simulink model "ModeInputHandle"  (R2018b)
settings: Solver=FixedStepDiscrete  StartTime=0.0  StopTime=10.0  FixedStep=0.01  RelTol=1e-3
undefined symbols (not defined in the file or in its folder): c, CmprtMdHMIReqExt2Tp1, CmprtMdHMIReqExtTp1, CmprtMdHMIReqTp1, d, e, EZESwReq1, f, g, IfVeSMSeStNumConfig, j, KeSMSuButtonLongPressedThrshldTm_Val, KeSMSuFoldType_Val, KeSMSwSeatSMSSeatMdTrigGapTimer_Val, KeSMSwSeatTrigWaitTimer_Val, KeSMSwSRSActiveValidTm_Val, LckUlckActvtFunc1, LstLckFunc1, LugSelectSw1, MdReqTp1, PowerMode1, SeatOccupiedSts1, SRSMode1, StPassCmprtMdCtrl_Md10_VCUConfig_Val, StPassCmprtMdCtrl_Md11_VCUConfig_Val, StPassCmprtMdCtrl_Md12_VCUConfig_Val, StPassCmprtMdCtrl_Md13_VCUConfig_Val, StPassCmprtMdCtrl_Md1_VCUConfig_Val, StPassCmprtMdCtrl_Md27_VCUConfig_Val, StPassCmprtMdCtrl_Md28_VCUConfig_Val, StPassCmprtMdCtrl_Md29_VCUConfig_Val, StPassCmprtMdCtrl_Md2_VCUConfig_Val, StPassCmprtMdCtrl_Md30_VCUConfig_Val, StPassCmprtMdCtrl_Md31_VCUConfig_Val, StPassCmprtMdCtrl_Md32_VCUConfig_Val, StPassCmprtMdCtrl_Md3_VCUConfig_Val, StPassCmprtMdCtrl_Md53_VCUConfig_Val, StPassCmprtMdCtrl_Md56_VCUConfig_Val, StPassCmprtMdCtrl_Md57_VCUConfig_Val, StPassCmprtMdCtrl_Md58_VCUConfig_Val, StPassCmprtMdCtrl_Md61_VCUConfig_Val, StPassCmprtMdCtrl_Md62_VCUConfig_Val, StPassCmprtMdCtrl_Md8_VCUConfig_Val, StPassCmprtMdCtrl_Md9_VCUConfig_Val, StSrv_StMd10_Config_Val, StSrv_StMd11_Config_Val, StSrv_StMd12_Config_Val, StSrv_StMd13_Config_Val, StSrv_StMd1_Config_Val, StSrv_StMd27_Config_Val, StSrv_StMd28_Config_Val, StSrv_StMd29_Config_Val, StSrv_StMd2_Config_Val, StSrv_StMd30_Config_Val, StSrv_StMd31_Config_Val, StSrv_StMd32_Config_Val, StSrv_StMd3_Config_Val, StSrv_StMd8_Config_Val, StSrv_StMd9_Config_Val, VehMovState1
libraries: MSMLib x91
(part 9 of 9)

== stateflow chart ModeInputHandle/ModelInputHandleRunnable_sys/Subsystem1/AcsEntry4s2RMdReq /ButtonLongPressed2/Chart1 ==
  state NotPressed
    en:
    oMdReq = false;
  state ButtonPressed
    state idle
    state idle1
      en:
      oMdReq = true;
    (default) -> idle
    idle -> idle1 : [after(iLongPressThrshhldTm,tick)]
  (default) -> NotPressed : {oMdInterruptCnt = 0;}
  NotPressed -> NotPressed [order 1] : [(iSRSMode != SRSCurMode1.SRSMode_None) &&...
      | hasChangedTo(iCnfmSwReq, true)]
      | {oMdInterruptCnt ++;}
  NotPressed -> ButtonPressed [order 2] : [iCurMdState == MdTp1.MdTp_None &&...
      | hasChangedTo(iSrc, true)]
  ButtonPressed -> NotPressed : [!iSrc]
  data: iSrc input boolean; oMdReq output boolean; oMdInterruptCnt output uint8; iLongPressThrshhldTm input uint8; iCurMdState input Enum: MdTp1; iCmpReq input; iCnfmSwReq input boolean; iSRSMode input Enum: SRSCurMode1

== stateflow chart ModeInputHandle/ModelInputHandleRunnable_sys/Subsystem1/AcsEntry4s2RMdReq /ButtonLongPressed/Chart1 ==
  state NotPressed
    en:
    oMdReq = false;
  state ButtonPressed
    state idle
      en:
      oMdInterruptCnt ++;
    state idle1
      en:
      oMdReq=true;
    (default) -> idle
    idle -> idle1 [order 1] : [after(iLongPressThrshhldTm,tick)]
  state wait
    en:
    oMdReq = false;
  (default) -> NotPressed : {oMdInterruptCnt = 0;}
  NotPressed -> ButtonPressed : [hasChangedTo(iSrc, true)]
  idle -> NotPressed [order 2] : [!iSrc]
  idle1 -> wait [order 2] : [after(5,tick)]
      | //[after(2,tick)]
  wait -> NotPressed : [!iSrc]
  idle1 -> NotPressed [order 1] : [!iSrc]
  data: iSrc input boolean; oMdReq output boolean; oMdInterruptCnt output uint8; iLongPressThrshhldTm input uint8

== stateflow chart ModeInputHandle/ModelInputHandleRunnable_sys/Subsystem1/AcsExit4s2RMdReq/ButtonLongPressed/Chart1 ==
  state NotPressed
    en:
    oMdReq = false;
  state ButtonPressed
    state idle
      en:
      oMdInterruptCnt ++;
    state idle1
      en:
      oMdReq=true;
    (default) -> idle
    idle -> idle1 [order 1] : [after(iLongPressThrshhldTm,tick)]
  state wait
    en:
    oMdReq = false;
  (default) -> NotPressed : {oMdInterruptCnt = 0;}
  NotPressed -> ButtonPressed : [hasChangedTo(iSrc, true)]
  idle -> NotPressed [order 2] : [!iSrc]
  idle1 -> wait [order 2] : [after(5,tick)]
      | //[after(2,tick)]
  wait -> NotPressed : [!iSrc]
  idle1 -> NotPressed [order 1] : [!iSrc]
  data: iSrc input boolean; oMdReq output boolean; oMdInterruptCnt output uint8; iLongPressThrshhldTm input uint8

== stateflow chart ModeInputHandle/ModelInputHandleRunnable_sys/Subsystem1/AcsExit4s2RMdReq/ButtonLongPressed2/Chart1 ==
  state NotPressed
    en:
    oMdReq = false;
  state ButtonPressed
    state idle
    state idle1
      en:
      oMdReq = true;
    (default) -> idle
    idle -> idle1 : [after(iLongPressThrshhldTm,tick)]
  (default) -> NotPressed : {oMdInterruptCnt = 0;}
  NotPressed -> NotPressed [order 1] : [(iSRSMode != SRSCurMode1.SRSMode_None) &&...
      | hasChangedTo(iCnfmSwReq, true)]
      | {oMdInterruptCnt ++;}
  NotPressed -> ButtonPressed [order 2] : [iCurMdState == MdTp1.MdTp_None &&...
      | hasChangedTo(iSrc, true)]
  ButtonPressed -> NotPressed : [!iSrc]
  data: iSrc input boolean; oMdReq output boolean; oMdInterruptCnt output uint8; iLongPressThrshhldTm input uint8; iCurMdState input Enum: MdTp1; iCmpReq input; iCnfmSwReq input boolean; iSRSMode input Enum: SRSCurMode1

== stateflow chart ModeInputHandle/ModelInputHandleRunnable_sys/Subsystem1/AcsEntryMdReq/ButtonLongPressed1/Chart1 ==
  state NotPressed
    en:
    oMdReq = false;
  state ButtonPressed
    state idle
      en:
      oMdInterruptCnt ++;
    state idle1
      en:
      oMdReq=true;
    (default) -> idle
    idle -> idle1 [order 1] : [after(iLongPressThrshhldTm,tick)]
  state wait
    en:
    oMdReq = false;
  (default) -> NotPressed : {oMdInterruptCnt = 0;}
  NotPressed -> ButtonPressed : [hasChangedTo(iSrc, true)]
  idle -> NotPressed [order 2] : [!iSrc]
  idle1 -> wait [order 2] : //[after(5,tick)]
      | [after(2,tick)]
  wait -> NotPressed : [!iSrc]
  idle1 -> NotPressed [order 1] : [!iSrc]
  data: iSrc input boolean; oMdReq output boolean; oMdInterruptCnt output uint8; iLongPressThrshhldTm input uint8

== stateflow chart ModeInputHandle/ModelInputHandleRunnable_sys/Subsystem1/AcsEntryAll4sBwdMdReq/Chart ==
  state UpdateOcclastStat [function]
    (default) -> (junction 55)
    (junction 55) -> (junction 57) [order 1] : [hasChanged(iNotSecRowLeSeaOccStat)]
    (junction 55) -> (junction 62) [order 2]
    (junction 57) -> (junction 59) : {iNotSecRowLeSeaOccStat_last = iNotSecRowLeSeaOccStat;}
    (junction 59) -> (junction 62)
    (junction 62) -> (junction 61)
    (junction 61) -> (junction 65) [order 1] : [hasChanged(iNotSecRowRtSeaOccStat)]
    (junction 61) -> (junction 70) [order 2]
    (junction 65) -> (junction 68) : {iNotSecRowRtSeaOccStat_last = iNotSecRowRtSeaOccStat;}
    (junction 68) -> (junction 70)
    (junction 70) -> (junction 73)
  state Wait1
    du:
    UpdateOcclastStat();
  state active
    en:
    oReq = true;
    iNotSecRowLeSeaOccStat_last = iNotSecRowLeSeaOccStat;
    iNotSecRowRtSeaOccStat_last = iNotSecRowRtSeaOccStat;
    du:
    UpdateOcclastStat();
  state inactive
    en:
    oReq = false;
    iNotSecRowLeSeaOccStat_last = iNotSecRowLeSeaOccStat;
    iNotSecRowRtSeaOccStat_last = iNotSecRowRtSeaOccStat;
    du:
    UpdateOcclastStat();
  state Wait2
    du:
    UpdateOcclastStat();
  (default) -> inactive
  inactive -> Wait1 [order 1] : [hasChangedTo(iRLDoorAjarSwAct,false)&&(iRRDoorAjarSwAct == false)]
  inactive -> Wait1 [order 2] : [hasChangedTo(iRRDoorAjarSwAct,false)&&(iRLDoorAjarSwAct == false)]
  Wait1 -> active [order 3] : [(((iNotSecRowLeSeaOccStat == SeatOccupiedSts1.SeatOccupiedSts_Occupied)&&...
      | (iNotSecRowLeSeaOccStat_last == SeatOccupiedSts1.SeatOccupiedSts_Empty))||...
      |  ((iNotSecRowRtSeaOccStat == SeatOccupiedSts1.SeatOccupiedSts_Occupied)&&...
      | (iNotSecRowRtSeaOccStat_last == SeatOccupiedSts1.SeatOccupiedSts_Empty)))]
  inactive -> Wait1 [order 4] : [hasChangedTo(iRLDoorAjarSwAct,false)&&hasChangedTo(iRRDoorAjarSwAct,false)]
  Wait1 -> inactive [order 1] : [after(iKeSMSwSeatSMSSeatMdTrigGapTimer,tick)]
  Wait1 -> inactive [order 2] : [(iRLDoorAjarSwAct == true)||(iRRDoorAjarSwAct == true)]
  Wait2 -> active [order 3] : [hasChangedTo(iRLDoorAjarSwAct,false) && (iRRDoorAjarSwAct == false)]
  Wait2 -> active [order 4] : [hasChangedTo(iRRDoorAjarSwAct,false) && (iRLDoorAjarSwAct == false)]
  inactive -> Wait2 [order 3] : [((iNotSecRowLeSeaOccStat == SeatOccupiedSts1.SeatOccupiedSts_Occupied)&&...
      | (iNotSecRowLeSeaOccStat_last == SeatOccupiedSts1.SeatOccupiedSts_Empty))||...
      |  ((iNotSecRowRtSeaOccStat == SeatOccupiedSts1.SeatOccupiedSts_Occupied)&&...
      | (iNotSecRowRtSeaOccStat_last == SeatOccupiedSts1.SeatOccupiedSts_Empty))]
  Wait2 -> active [order 5] : [hasChangedTo(iRLDoorAjarSwAct,false)&&hasChangedTo(iRRDoorAjarSwAct,false)]
  Wait2 -> inactive [order 1] : [after(iKeSMSwSeatSMSSeatMdTrigGapTimer,tick)]
  Wait2 -> inactive [order 2] : [(iNotSecRowLeSeaOccStat == SeatOccupiedSts1.SeatOccupiedSts_Empty)&&...
      | (iNotSecRowRtSeaOccStat == SeatOccupiedSts1.SeatOccupiedSts_Empty)]
  active -> inactive : [after(3,tick)]
  data: oReq output boolean; iRLDoorAjarSwAct input boolean; iRRDoorAjarSwAct input boolean; iKeSMSwSeatSMSSeatMdTrigGapTimer input uint16; iNotSecRowLeSeaOccStat input Enum: SeatOccupiedSts1; iNotSecRowRtSeaOccStat input Enum: SeatOccupiedSts1; iNotSecRowLeSeaOccStat_last local Enum: SeatOccupiedSts1 size=1; iNotSecRowRtSeaOccStat_last local Enum: SeatOccupiedSts1 size=1; flag local uint8 size=1

== stateflow chart ModeInputHandle/ModelInputHandleRunnable_sys/Subsystem1/AcsEntryAll4sFwdMdReq/Chart ==
  state Init
    en:
    AcsEntryAll4sFwdMdV = false;
  state WaitOccSign
    en:
    AcsEntryAll4sFwdMdV = false;
  state MdAvail
    en:
    AcsEntryAll4sFwdMdV = true;
  (default) -> Init
  WaitOccSign -> Init [order 2] : [after(iKeSMSwSeatTrigWaitTimer,tick)]
  (junction 34) -> WaitOccSign [order 2]
  WaitOccSign -> MdAvail [order 1] : [(ibVehMovState == true) && (ibSysPwrMd == true) &&...
      | (ibNotSecRowLRSeaOccEmpty == true)]
  Init -> (junction 34) : [(ibLstLckFunc == true) && (ibLstLckChange == true) &&...
      |  (ibLckUlckActvtFunc == true)]
  (junction 34) -> MdAvail [order 1] : [(ibVehMovState == true) && (ibSysPwrMd == true) &&...
      | (ibNotSecRowLRSeaOccEmpty == true)]
  MdAvail -> Init : [(ibVehMovState == false) || (ibSysPwrMd == false) ||...
      |  (ibLstLckFunc == false) || (ibLstLckChange == false) ||...
      |  (ibLckUlckActvtFunc == false) || (ibNotSecRowLRSeaOccEmpty == false)]
  data: ibVehMovState input; ibSysPwrMd input; ibLstLckFunc input; ibLstLckChange input; ibLckUlckActvtFunc input; ibNotSecRowLRSeaOccEmpty input; iKeSMSwSeatTrigWaitTimer input; AcsEntryAll4sFwdMdV output boolean

== stateflow chart ModeInputHandle/ModelInputHandleRunnable_sys/Subsystem1/PasReclinerEntryMdReq/ButtonLongPressed/Chart1 ==
  state NotPressed
    en:
    oMdReq = false;
  state ButtonPressed
    state idle
      en:
      oMdInterruptCnt ++;
    state idle1
      en:
      oMdReq=true;
    (default) -> idle
    idle -> idle1 [order 1] : [after(iLongPressThrshhldTm,tick)]
  state wait
    en:
    oMdReq = false;
  (default) -> NotPressed : {oMdInterruptCnt = 0;}
  NotPressed -> ButtonPressed : [hasChangedTo(iSrc, true)]
  idle -> NotPressed [order 2] : [!iSrc]
  wait -> NotPressed : [!iSrc]
  idle1 -> wait [order 2] : //[after(5,tick)]
      | [after(2,tick)]
  idle1 -> NotPressed [order 1] : [!iSrc]
  data: iSrc input boolean; oMdReq output boolean; oMdInterruptCnt output uint8; iLongPressThrshhldTm input uint8

== stateflow chart ModeInputHandle/ModelInputHandleRunnable_sys/Subsystem1/PasReclinerExitMdReq/ButtonLongPressed/Chart1 ==
  state NotPressed
    en:
    oMdReq = false;
  state ButtonPressed
    state idle
      en:
      oMdInterruptCnt ++;
    state idle1
      en:
      oMdReq=true;
    (default) -> idle
    idle -> idle1 [order 1] : [after(iLongPressThrshhldTm,tick)]
  state wait
    en:
    oMdReq = false;
  (default) -> NotPressed : {oMdInterruptCnt = 0;}
  NotPressed -> ButtonPressed : [hasChangedTo(iSrc, true)]
  idle -> NotPressed [order 2] : [!iSrc]
  wait -> NotPressed : [!iSrc]
  idle1 -> wait [order 2] : //[after(5,tick)]
      | [after(2,tick)]
  idle1 -> NotPressed [order 1] : [!iSrc]
  data: iSrc input boolean; oMdReq output boolean; oMdInterruptCnt output uint8; iLongPressThrshhldTm input uint8

== stateflow chart ModeInputHandle/ModelInputHandleRunnable_sys/Subsystem1/UnfoldMdReq/ButtonLongPressed/Chart1 ==
  state NotPressed
    en:
    oMdReq = false;
  state ButtonPressed
    state idle
      en:
      oMdInterruptCnt ++;
    state idle1
      en:
      oMdReq=true;
    (default) -> idle
    idle -> idle1 [order 1] : [after(iLongPressThrshhldTm,tick)]
  state wait
    en:
    oMdReq = false;
  (default) -> NotPressed : {oMdInterruptCnt = 0;}
  NotPressed -> ButtonPressed : [hasChangedTo(iSrc, true)]
  idle -> NotPressed [order 2] : [!iSrc]
  wait -> NotPressed : [!iSrc]
  idle1 -> wait [order 2] : //[after(5,tick)]
      | [after(2,tick)]
  idle1 -> NotPressed [order 1] : [!iSrc]
  data: iSrc input boolean; oMdReq output boolean; oMdInterruptCnt output uint8; iLongPressThrshhldTm input uint8

== stateflow chart ModeInputHandle/ModelInputHandleRunnable_sys/Subsystem1/UnfoldMdReq/ButtonLongPressed1/Chart1 ==
  state NotPressed
    en:
    oMdReq = false;
  state ButtonPressed
    state idle
      en:
      oMdInterruptCnt ++;
    state idle1
      en:
      oMdReq=true;
    (default) -> idle
    idle -> idle1 [order 1] : [after(iLongPressThrshhldTm,tick)]
  state wait
    en:
    oMdReq = false;
  (default) -> NotPressed : {oMdInterruptCnt = 0;}
  NotPressed -> ButtonPressed : [hasChangedTo(iSrc, true)]
  idle -> NotPressed [order 2] : [!iSrc]
  wait -> NotPressed : [!iSrc]
  idle1 -> wait [order 2] : //[after(5,tick)]
      | [after(2,tick)]
  idle1 -> NotPressed [order 1] : [!iSrc]
  data: iSrc input boolean; oMdReq output boolean; oMdInterruptCnt output uint8; iLongPressThrshhldTm input uint8

== stateflow chart ModeInputHandle/ModelInputHandleRunnable_sys/Subsystem1/AcsEntryMdReq/ButtonLongPressed4/Chart1 ==
  state NotPressed
    en:
    oMdReq = false;
  state ButtonPressed
    state idle
      en:
      oMdInterruptCnt ++;
    state idle1
      en:
      oMdReq=true;
    (default) -> idle
    idle -> idle1 [order 1] : [after(iLongPressThrshhldTm,tick)]
  state wait
    en:
    oMdReq = false;
  (default) -> NotPressed : {oMdInterruptCnt = 0;}
  NotPressed -> ButtonPressed : [hasChangedTo(iSrc, true)]
  idle -> NotPressed [order 2] : [!iSrc]
  idle1 -> wait [order 2] : //[after(5,tick)]
      | [after(2,tick)]
  wait -> NotPressed : [!iSrc]
  idle1 -> NotPressed [order 1] : [!iSrc]
  data: iSrc input boolean; oMdReq output boolean; oMdInterruptCnt output uint8; iLongPressThrshhldTm input uint8

== stateflow chart ModeInputHandle/ModelInputHandleRunnable_sys/Subsystem1/AcsEntryMdReq/ButtonLongPressed2/Chart1 ==
  state NotPressed
    en:
    oMdReq = false;
  state ButtonPressed
    state idle
    state idle1
      en:
      oMdReq = true;
    (default) -> idle
    idle -> idle1 : [after(iLongPressThrshhldTm,tick)]
  (default) -> NotPressed : {oMdInterruptCnt = 0;}
  NotPressed -> NotPressed [order 1] : [(iSRSMode != SRSCurMode1.SRSMode_None) &&...
      | hasChangedTo(iCnfmSwReq, true)]
      | {oMdInterruptCnt ++;}
  NotPressed -> ButtonPressed [order 2] : [iCurMdState == MdTp1.MdTp_None &&...
      | hasChangedTo(iSrc, true)]
  ButtonPressed -> NotPressed : [!iSrc]
  data: iSrc input boolean; oMdReq output boolean; oMdInterruptCnt output uint8; iLongPressThrshhldTm input uint8; iCurMdState input Enum: MdTp1; iCmpReq input; iCnfmSwReq input boolean; iSRSMode input Enum: SRSCurMode1

== stateflow chart ModeInputHandle/ModelInputHandleRunnable_sys/Subsystem1/AcsEntryMdReq/ButtonLongPressed3/Chart1 ==
  state NotPressed
    en:
    oMdReq = false;
  state ButtonPressed
    state idle
      en:
      oMdInterruptCnt ++;
    state idle1
      en:
      oMdReq=true;
    (default) -> idle
    idle -> idle1 [order 1] : [after(iLongPressThrshhldTm,tick)]
  state wait
    en:
    oMdReq = false;
  (default) -> NotPressed : {oMdInterruptCnt = 0;}
  NotPressed -> ButtonPressed : [hasChangedTo(iSrc, true)]
  idle -> NotPressed [order 2] : [!iSrc]
  wait -> NotPressed : [!iSrc]
  idle1 -> wait [order 2] : //[after(5,tick)]
      | [after(2,tick)]
  idle1 -> NotPressed [order 1] : [!iSrc]
  data: iSrc input boolean; oMdReq output boolean; oMdInterruptCnt output uint8; iLongPressThrshhldTm input uint8

== stateflow chart ModeInputHandle/ModelInputHandleRunnable_sys/Subsystem1/AcsExtMdReq/ButtonLongPressed/Chart1 ==
  state ButtonPressed
    state idle
      en:
      oMdInterruptCnt ++;
    state idle1
      en:
      oMdReq=true;
    (default) -> idle
    idle -> idle1 [order 1] : [after(iLongPressThrshhldTm,tick)]
  state NotPressed
    en:
    oMdReq = false;
  state wait
    en:
    oMdReq = false;
  (default) -> NotPressed : {oMdInterruptCnt = 0;}
  NotPressed -> ButtonPressed : [hasChangedTo(iSrc, true)]
  idle -> NotPressed [order 2] : [!iSrc]
  idle1 -> wait [order 2] : [after(5,tick)]
      | //[after(2,tick)]
  wait -> NotPressed : [!iSrc]
  idle1 -> NotPressed [order 1] : [!iSrc]
  data: iSrc input boolean; oMdReq output boolean; oMdInterruptCnt output uint8; iLongPressThrshhldTm input uint8

== stateflow chart ModeInputHandle/ModelInputHandleRunnable_sys/Subsystem1/AcsExtMdReq/ButtonLongPressed1/Chart1 ==
  state NotPressed
    en:
    oMdReq = false;
  state ButtonPressed
    state idle
      en:
      oMdInterruptCnt ++;
    state idle1
      en:
      oMdReq=true;
    (default) -> idle
    idle -> idle1 [order 1] : [after(iLongPressThrshhldTm,tick)]
  state wait
    en:
    oMdReq = false;
  (default) -> NotPressed : {oMdInterruptCnt = 0;}
  NotPressed -> ButtonPressed : [hasChangedTo(iSrc, true)]
  idle -> NotPressed [order 2] : [!iSrc]
  idle1 -> wait [order 2] : [after(5,tick)]
      | //[after(2,tick)]
  wait -> NotPressed : [!iSrc]
  idle1 -> NotPressed [order 1] : [!iSrc]
  data: iSrc input boolean; oMdReq output boolean; oMdInterruptCnt output uint8; iLongPressThrshhldTm input uint8

== stateflow chart ModeInputHandle/ModelInputHandleRunnable_sys/Subsystem1/AcsExtMdReq/ButtonLongPressed2/Chart1 ==
  state NotPressed
    en:
    oMdReq = false;
  state ButtonPressed
    state idle
    state idle1
      en:
      oMdReq = true;
    (default) -> idle
    idle -> idle1 : [after(iLongPressThrshhldTm,tick)]
  (default) -> NotPressed : {oMdInterruptCnt = 0;}
  NotPressed -> NotPressed [order 1] : [(iSRSMode != SRSCurMode1.SRSMode_None) &&...
      | hasChangedTo(iCnfmSwReq, true)]
      | {oMdInterruptCnt ++;}
  NotPressed -> ButtonPressed [order 2] : [iCurMdState == MdTp1.MdTp_None &&...
      | hasChangedTo(iSrc, true)]
  ButtonPressed -> NotPressed : [!iSrc]
  data: iSrc input boolean; oMdReq output boolean; oMdInterruptCnt output uint8; iLongPressThrshhldTm input uint8; iCurMdState input Enum: MdTp1; iCmpReq input; iCnfmSwReq input boolean; iSRSMode input Enum: SRSCurMode1

== stateflow chart ModeInputHandle/ModelInputHandleRunnable_sys/Subsystem1/FamilyMdReq/ButtonLongPressed2/Chart1 ==
  state NotPressed
    en:
    oMdReq = false;
  state ButtonPressed
    state idle
    state idle1
      en:
      oMdReq = true;
    (default) -> idle
    idle -> idle1 : [after(iLongPressThrshhldTm,tick)]
  (default) -> NotPressed : {oMdInterruptCnt = 0;}
  NotPressed -> NotPressed [order 1] : [(iSRSMode != SRSMode1.SRSSlctSwStat_None) &&...
      | hasChangedTo(iCnfmSwReq, true)]
      | {oMdInterruptCnt ++;}
  NotPressed -> ButtonPressed [order 2] : [iCurMdState == MdTp1.MdTp_None &&...
      | hasChangedTo(iSrc, true)]
  ButtonPressed -> NotPressed : [!iSrc]
  data: iSrc input boolean; oMdReq output boolean; oMdInterruptCnt output uint8; iLongPressThrshhldTm input uint8; iCurMdState input Enum: MdTp1; iCmpReq input; iCnfmSwReq input boolean; iSRSMode input Enum: SRSCurMode1

== stateflow chart ModeInputHandle/ModelInputHandleRunnable_sys/Subsystem1/FamilyMdReq/ButtonLongPressed4/Chart1 ==
  state NotPressed
    en:
    oMdReq = false;
  state ButtonPressed
    state idle
    state idle1
      en:
      oMdReq = true;
    (default) -> idle
    idle -> idle1 : [after(iLongPressThrshhldTm,tick)]
  (default) -> NotPressed : {oMdInterruptCnt = 0;}
  NotPressed -> NotPressed [order 1] : [(iSRSMode != SRSMode1.SRSSlctSwStat_None) &&...
      | hasChangedTo(iCnfmSwReq, true)]
      | {oMdInterruptCnt ++;}
  NotPressed -> ButtonPressed [order 2] : [iCurMdState == MdTp1.MdTp_None &&...
      | hasChangedTo(iSrc, true)]
  ButtonPressed -> NotPressed : [!iSrc]
  data: iSrc input boolean; oMdReq output boolean; oMdInterruptCnt output uint8; iLongPressThrshhldTm input uint8; iCurMdState input Enum: MdTp1; iCmpReq input; iCnfmSwReq input boolean; iSRSMode input Enum: SRSCurMode1

== stateflow chart ModeInputHandle/ModelInputHandleRunnable_sys/Subsystem1/IntimacyReq/ButtonLongPressed1/Chart1 ==
  state NotPressed
    en:
    oMdReq = false;
  state ButtonPressed
    state idle
    state idle1
      en:
      oMdReq = true;
    (default) -> idle
    idle -> idle1 : [after(iLongPressThrshhldTm,tick)]
  (default) -> NotPressed : {oMdInterruptCnt = 0;}
  NotPressed -> NotPressed [order 1] : [(iSRSMode != SRSMode1.SRSSlctSwStat_None) &&...
      | hasChangedTo(iCnfmSwReq, true)]
      | {oMdInterruptCnt ++;}
  NotPressed -> ButtonPressed [order 2] : [iCurMdState == MdTp1.MdTp_None &&...
      | hasChangedTo(iSrc, true)]
  ButtonPressed -> NotPressed : [!iSrc]
  data: iSrc input boolean; oMdReq output boolean; oMdInterruptCnt output uint8; iLongPressThrshhldTm input uint8; iCurMdState input Enum: MdTp1; iCmpReq input; iCnfmSwReq input boolean; iSRSMode input Enum: SRSCurMode1

== stateflow chart ModeInputHandle/ModelInputHandleRunnable_sys/Subsystem1/IntimacyReq/ButtonLongPressed4/Chart1 ==
  state NotPressed
    en:
    oMdReq = false;
  state ButtonPressed
    state idle
    state idle1
      en:
      oMdReq = true;
    (default) -> idle
    idle -> idle1 : [after(iLongPressThrshhldTm,tick)]
  (default) -> NotPressed : {oMdInterruptCnt = 0;}
  NotPressed -> NotPressed [order 1] : [(iSRSMode != SRSMode1.SRSSlctSwStat_None) &&...
      | hasChangedTo(iCnfmSwReq, true)]
      | {oMdInterruptCnt ++;}
  NotPressed -> ButtonPressed [order 2] : [iCurMdState == MdTp1.MdTp_None &&...
      | hasChangedTo(iSrc, true)]
  ButtonPressed -> NotPressed : [!iSrc]
  data: iSrc input boolean; oMdReq output boolean; oMdInterruptCnt output uint8; iLongPressThrshhldTm input uint8; iCurMdState input Enum: MdTp1; iCmpReq input; iCnfmSwReq input boolean; iSRSMode input Enum: SRSCurMode1

== stateflow chart ModeInputHandle/ModelInputHandleRunnable_sys/Subsystem1/LgrstLtMdReq/ButtonLongPressed2/Chart1 ==
  state NotPressed
    en:
    oMdReq = false;
  state ButtonPressed
    state idle
    state idle1
      en:
      oMdReq = true;
    (default) -> idle
    idle -> idle1 : [after(iLongPressThrshhldTm,tick)]
  (default) -> NotPressed : {oMdInterruptCnt = 0;}
  NotPressed -> NotPressed [order 1] : [(iSRSMode != SRSMode1.SRSSlctSwStat_None) &&...
      | hasChangedTo(iCnfmSwReq, true)]
      | {oMdInterruptCnt ++;}
  NotPressed -> ButtonPressed [order 2] : [iCurMdState == MdTp1.MdTp_None &&...
      | hasChangedTo(iSrc, true)]
  ButtonPressed -> NotPressed : [!iSrc]
  data: iSrc input boolean; oMdReq output boolean; oMdInterruptCnt output uint8; iLongPressThrshhldTm input uint8; iCurMdState input Enum: MdTp1; iCmpReq input; iCnfmSwReq input boolean; iSRSMode input Enum: SRSCurMode1

== stateflow chart ModeInputHandle/ModelInputHandleRunnable_sys/Subsystem1/LgrstLtMdReq/ButtonLongPressed4/Chart1 ==
  state NotPressed
    en:
    oMdReq = false;
  state ButtonPressed
    state idle
    state idle1
      en:
      oMdReq = true;
    (default) -> idle
    idle -> idle1 : [after(iLongPressThrshhldTm,tick)]
  (default) -> NotPressed : {oMdInterruptCnt = 0;}
  NotPressed -> NotPressed [order 1] : [(iSRSMode != SRSMode1.SRSSlctSwStat_None) &&...
      | hasChangedTo(iCnfmSwReq, true)]
      | {oMdInterruptCnt ++;}
  NotPressed -> ButtonPressed [order 2] : [iCurMdState == MdTp1.MdTp_None &&...
      | hasChangedTo(iSrc, true)]
  ButtonPressed -> NotPressed : [!iSrc]
  data: iSrc input boolean; oMdReq output boolean; oMdInterruptCnt output uint8; iLongPressThrshhldTm input uint8; iCurMdState input Enum: MdTp1; iCmpReq input; iCnfmSwReq input boolean; iSRSMode input Enum: SRSCurMode1

== stateflow chart ModeInputHandle/ModelInputHandleRunnable_sys/Subsystem1/LgrstRtMdReq/ButtonLongPressed2/Chart1 ==
  state NotPressed
    en:
    oMdReq = false;
  state ButtonPressed
    state idle
    state idle1
      en:
      oMdReq = true;
    (default) -> idle
    idle -> idle1 : [after(iLongPressThrshhldTm,tick)]
  (default) -> NotPressed : {oMdInterruptCnt = 0;}
  NotPressed -> NotPressed [order 1] : [(iSRSMode != SRSMode1.SRSSlctSwStat_None) &&...
      | hasChangedTo(iCnfmSwReq, true)]
      | {oMdInterruptCnt ++;}
  NotPressed -> ButtonPressed [order 2] : [iCurMdState == MdTp1.MdTp_None &&...
      | hasChangedTo(iSrc, true)]
  ButtonPressed -> NotPressed : [!iSrc]
  data: iSrc input boolean; oMdReq output boolean; oMdInterruptCnt output uint8; iLongPressThrshhldTm input uint8; iCurMdState input Enum: MdTp1; iCmpReq input; iCnfmSwReq input boolean; iSRSMode input Enum: SRSCurMode1

== stateflow chart ModeInputHandle/ModelInputHandleRunnable_sys/Subsystem1/LgrstRtMdReq/ButtonLongPressed4/Chart1 ==
  state NotPressed
    en:
    oMdReq = false;
  state ButtonPressed
    state idle
    state idle1
      en:
      oMdReq = true;
    (default) -> idle
    idle -> idle1 : [after(iLongPressThrshhldTm,tick)]
  (default) -> NotPressed : {oMdInterruptCnt = 0;}
  NotPressed -> NotPressed [order 1] : [(iSRSMode != SRSMode1.SRSSlctSwStat_None) &&...
      | hasChangedTo(iCnfmSwReq, true)]
      | {oMdInterruptCnt ++;}
  NotPressed -> ButtonPressed [order 2] : [iCurMdState == MdTp1.MdTp_None &&...
      | hasChangedTo(iSrc, true)]
  ButtonPressed -> NotPressed : [!iSrc]
  data: iSrc input boolean; oMdReq output boolean; oMdInterruptCnt output uint8; iLongPressThrshhldTm input uint8; iCurMdState input Enum: MdTp1; iCmpReq input; iCnfmSwReq input boolean; iSRSMode input Enum: SRSCurMode1

== stateflow chart ModeInputHandle/ModelInputHandleRunnable_sys/Subsystem1/LugMdReq/ButtonLongPressed/Chart1 ==
  state NotPressed
    en:
    oMdReq = false;
  state ButtonPressed
    state idle
      en:
      oMdInterruptCnt ++;
    state idle1
      en:
      oMdReq=true;
    (default) -> idle
    idle -> idle1 [order 1] : [after(iLongPressThrshhldTm,tick)]
  state wait
    en:
    oMdReq = false;
  (default) -> NotPressed : {oMdInterruptCnt = 0;}
  NotPressed -> ButtonPressed : [hasChangedTo(iSrc, true)]
  idle -> NotPressed [order 2] : [!iSrc]
  wait -> NotPressed : [!iSrc]
  idle1 -> wait [order 2] : //[after(5,tick)]
      | [after(2,tick)]
  idle1 -> NotPressed [order 1] : [!iSrc]
  data: iSrc input boolean; oMdReq output boolean; oMdInterruptCnt output uint8; iLongPressThrshhldTm input uint8

== stateflow chart ModeInputHandle/ModelInputHandleRunnable_sys/Subsystem1/LugMdReq/ButtonLongPressed1/Chart1 ==
  state NotPressed
    en:
    oMdReq = false;
  state ButtonPressed
    state idle
      en:
      oMdInterruptCnt ++;
    state idle1
      en:
      oMdReq=true;
    (default) -> idle
    idle -> idle1 [order 1] : [after(iLongPressThrshhldTm,tick)]
  state wait
    en:
    oMdReq = false;
  (default) -> NotPressed : {oMdInterruptCnt = 0;}
  NotPressed -> ButtonPressed : [hasChangedTo(iSrc, true)]
  idle -> NotPressed [order 2] : [!iSrc]
  idle1 -> wait [order 2] : //[after(5,tick)]
      | [after(2,tick)]
  wait -> NotPressed : [!iSrc]
  idle1 -> NotPressed [order 1] : [!iSrc]
  data: iSrc input boolean; oMdReq output boolean; oMdInterruptCnt output uint8; iLongPressThrshhldTm input uint8

== stateflow chart ModeInputHandle/ModelInputHandleRunnable_sys/Subsystem1/LugMdReq/ButtonLongPressed2/Chart1 ==
  state NotPressed
    en:
    oMdReq = false;
  state ButtonPressed
    state idle
      en:
      oMdInterruptCnt ++;
    state idle1
      en:
      oMdReq=true;
    (default) -> idle
    idle -> idle1 [order 1] : [after(iLongPressThrshhldTm,tick)]
  state wait
    en:
    oMdReq = false;
  (default) -> NotPressed : {oMdInterruptCnt = 0;}
  NotPressed -> ButtonPressed : [hasChangedTo(iSrc, true)]
  idle -> NotPressed [order 2] : [!iSrc]
  wait -> NotPressed : [!iSrc]
  idle1 -> wait [order 2] : //[after(5,tick)]
      | [after(2,tick)]
  idle1 -> NotPressed [order 1] : [!iSrc]
  data: iSrc input boolean; oMdReq output boolean; oMdInterruptCnt output uint8; iLongPressThrshhldTm input uint8

== stateflow chart ModeInputHandle/ModelInputHandleRunnable_sys/Subsystem1/LugMdReq/ButtonLongPressed3/Chart1 ==
  state NotPressed
    en:
    oMdReq = false;
  state ButtonPressed
    state idle
    state idle1
      en:
      oMdReq = true;
    (default) -> idle
    idle -> idle1 : [after(iLongPressThrshhldTm,tick)]
  (default) -> NotPressed : {oMdInterruptCnt = 0;}
  NotPressed -> NotPressed [order 1] : [(iSRSMode != SRSMode1.SRSSlctSwStat_None) &&...
      | hasChangedTo(iCnfmSwReq, true)]
      | {oMdInterruptCnt ++;}
  NotPressed -> ButtonPressed [order 2] : [iCurMdState == MdTp1.MdTp_None &&...
      | hasChangedTo(iSrc, true)]
  ButtonPressed -> NotPressed : [!iSrc]
  data: iSrc input boolean; oMdReq output boolean; oMdInterruptCnt output uint8; iLongPressThrshhldTm input uint8; iCurMdState input Enum: MdTp1; iCmpReq input; iCnfmSwReq input boolean; iSRSMode input Enum: SRSCurMode1

== stateflow chart ModeInputHandle/ModelInputHandleRunnable_sys/Subsystem1/LugMdReq/ButtonLongPressed4/Chart1 ==
  state NotPressed
    en:
    oMdReq = false;
  state ButtonPressed
    state idle
    state idle1
      en:
      oMdReq = true;
    (default) -> idle
    idle -> idle1 : [after(iLongPressThrshhldTm,tick)]
  (default) -> NotPressed : {oMdInterruptCnt = 0;}
  NotPressed -> NotPressed [order 1] : [(iSRSMode != SRSMode1.SRSSlctSwStat_None) &&...
      | hasChangedTo(iCnfmSwReq, true)]
      | {oMdInterruptCnt ++;}
  NotPressed -> ButtonPressed [order 2] : [iCurMdState == MdTp1.MdTp_None &&...
      | hasChangedTo(iSrc, true)]
  ButtonPressed -> NotPressed : [!iSrc]
  data: iSrc input boolean; oMdReq output boolean; oMdInterruptCnt output uint8; iLongPressThrshhldTm input uint8; iCurMdState input Enum: MdTp1; iCmpReq input; iCnfmSwReq input boolean; iSRSMode input Enum: SRSCurMode1

== stateflow chart ModeInputHandle/ModelInputHandleRunnable_sys/Subsystem1/LugMdReq/ButtonLongPressed5/Chart1 ==
  state NotPressed
    en:
    oMdReq = false;
  state ButtonPressed
    state idle
    state idle1
      en:
      oMdReq = true;
    (default) -> idle
    idle -> idle1 : [after(iLongPressThrshhldTm,tick)]
  (default) -> NotPressed : {oMdInterruptCnt = 0;}
  NotPressed -> NotPressed [order 1] : [(iSRSMode != SRSMode1.SRSSlctSwStat_None) &&...
      | hasChangedTo(iCnfmSwReq, true)]
      | {oMdInterruptCnt ++;}
  NotPressed -> ButtonPressed [order 2] : [iCurMdState == MdTp1.MdTp_None &&...
      | hasChangedTo(iSrc, true)]
  ButtonPressed -> NotPressed : [!iSrc]
  data: iSrc input boolean; oMdReq output boolean; oMdInterruptCnt output uint8; iLongPressThrshhldTm input uint8; iCurMdState input Enum: MdTp1; iCmpReq input; iCnfmSwReq input boolean; iSRSMode input Enum: SRSCurMode1

== stateflow chart ModeInputHandle/ModelInputHandleRunnable_sys/Subsystem1/LugMdReq/ButtonLongPressed6/Chart1 ==
  state NotPressed
    en:
    oMdReq = false;
  state ButtonPressed
    state idle
      en:
      oMdInterruptCnt ++;
    state idle1
      en:
      oMdReq=true;
    (default) -> idle
    idle -> idle1 [order 1] : [after(iLongPressThrshhldTm,tick)]
  state wait
    en:
    oMdReq = false;
  (default) -> NotPressed : {oMdInterruptCnt = 0;}
  NotPressed -> ButtonPressed : [hasChangedTo(iSrc, true)]
  idle -> NotPressed [order 2] : [!iSrc]
  wait -> NotPressed : [!iSrc]
  idle1 -> wait [order 2] : //[after(5,tick)]
      | [after(2,tick)]
  idle1 -> NotPressed [order 1] : [!iSrc]
  data: iSrc input boolean; oMdReq output boolean; oMdInterruptCnt output uint8; iLongPressThrshhldTm input uint8

== stateflow chart ModeInputHandle/ModelInputHandleRunnable_sys/Subsystem1/LyingMdReq/ButtonLongPressed2/Chart1 ==
  state NotPressed
    en:
    oMdReq = false;
  state ButtonPressed
    state idle
    state idle1
      en:
      oMdReq = true;
    (default) -> idle
    idle -> idle1 : [after(iLongPressThrshhldTm,tick)]
  (default) -> NotPressed : {oMdInterruptCnt = 0;}
  NotPressed -> NotPressed [order 1] : [(iSRSMode != SRSMode1.SRSSlctSwStat_None) &&...
      | hasChangedTo(iCnfmSwReq, true)]
      | {oMdInterruptCnt ++;}
  NotPressed -> ButtonPressed [order 2] : [iCurMdState == MdTp1.MdTp_None &&...
      | hasChangedTo(iSrc, true)]
  ButtonPressed -> NotPressed : [!iSrc]
  data: iSrc input boolean; oMdReq output boolean; oMdInterruptCnt output uint8; iLongPressThrshhldTm input uint8; iCurMdState input Enum: MdTp1; iCmpReq input; iCnfmSwReq input boolean; iSRSMode input Enum: SRSCurMode1

== stateflow chart ModeInputHandle/ModelInputHandleRunnable_sys/Subsystem1/LyingMdReq/ButtonLongPressed4/Chart1 ==
  state NotPressed
    en:
    oMdReq = false;
  state ButtonPressed
    state idle
    state idle1
      en:
      oMdReq = true;
    (default) -> idle
    idle -> idle1 : [after(iLongPressThrshhldTm,tick)]
  (default) -> NotPressed : {oMdInterruptCnt = 0;}
  NotPressed -> NotPressed [order 1] : [(iSRSMode != SRSMode1.SRSSlctSwStat_None) &&...
      | hasChangedTo(iCnfmSwReq, true)]
      | {oMdInterruptCnt ++;}
  NotPressed -> ButtonPressed [order 2] : [iCurMdState == MdTp1.MdTp_None &&...
      | hasChangedTo(iSrc, true)]
  ButtonPressed -> NotPressed : [!iSrc]
  data: iSrc input boolean; oMdReq output boolean; oMdInterruptCnt output uint8; iLongPressThrshhldTm input uint8; iCurMdState input Enum: MdTp1; iCmpReq input; iCnfmSwReq input boolean; iSRSMode input Enum: SRSCurMode1

== stateflow chart ModeInputHandle/ModelInputHandleRunnable_sys/Subsystem1/RecoveryMdReq/ButtonLongPressed/Chart1 ==
  state NotPressed
    en:
    oMdReq = false;
  state ButtonPressed
    state idle
      en:
      oMdInterruptCnt ++;
    state idle1
      en:
      oMdReq=true;
    (default) -> idle
    idle -> idle1 [order 1] : [after(iLongPressThrshhldTm,tick)]
  state wait
    en:
    oMdReq = false;
  (default) -> NotPressed : {oMdInterruptCnt = 0;}
  NotPressed -> ButtonPressed : [hasChangedTo(iSrc, true)]
  idle -> NotPressed [order 2] : [!iSrc]
  wait -> NotPressed : [!iSrc]
  idle1 -> wait [order 2] : //[after(5,tick)]
      | [after(2,tick)]
  idle1 -> NotPressed [order 1] : [!iSrc]
  data: iSrc input boolean; oMdReq output boolean; oMdInterruptCnt output uint8; iLongPressThrshhldTm input uint8

== stateflow chart ModeInputHandle/ModelInputHandleRunnable_sys/Subsystem1/RecoveryMdReq/ButtonLongPressed1/Chart1 ==
  state NotPressed
    en:
    oMdReq = false;
  state ButtonPressed
    state idle
      en:
      oMdInterruptCnt ++;
    state idle1
      en:
      oMdReq=true;
    (default) -> idle
    idle -> idle1 [order 1] : [after(iLongPressThrshhldTm,tick)]
  state wait
    en:
    oMdReq = false;
  (default) -> NotPressed : {oMdInterruptCnt = 0;}
  NotPressed -> ButtonPressed : [hasChangedTo(iSrc, true)]
  idle -> NotPressed [order 2] : [!iSrc]
  wait -> NotPressed : [!iSrc]
  idle1 -> wait [order 2] : //[after(5,tick)]
      | [after(2,tick)]
  idle1 -> NotPressed [order 1] : [!iSrc]
  data: iSrc input boolean; oMdReq output boolean; oMdInterruptCnt output uint8; iLongPressThrshhldTm input uint8

== stateflow chart ModeInputHandle/ModelInputHandleRunnable_sys/Subsystem1/RecoveryMdReq/ButtonLongPressed2/Chart1 ==
  state NotPressed
    en:
    oMdReq = false;
  state ButtonPressed
    state idle
    state idle1
      en:
      oMdReq = true;
    (default) -> idle
    idle -> idle1 : [after(iLongPressThrshhldTm,tick)]
  (default) -> NotPressed : {oMdInterruptCnt = 0;}
  NotPressed -> NotPressed [order 1] : [(iSRSMode != SRSMode1.SRSSlctSwStat_None) &&...
      | hasChangedTo(iCnfmSwReq, true)]
      | {oMdInterruptCnt ++;}
  NotPressed -> ButtonPressed [order 2] : [iCurMdState == MdTp1.MdTp_None &&...
      | hasChangedTo(iSrc, true)]
  ButtonPressed -> NotPressed : [!iSrc]
  data: iSrc input boolean; oMdReq output boolean; oMdInterruptCnt output uint8; iLongPressThrshhldTm input uint8; iCurMdState input Enum: MdTp1; iCmpReq input; iCnfmSwReq input boolean; iSRSMode input Enum: SRSCurMode1

== stateflow chart ModeInputHandle/ModelInputHandleRunnable_sys/Subsystem1/RecoveryMdReq/ButtonLongPressed4/Chart1 ==
  state NotPressed
    en:
    oMdReq = false;
  state ButtonPressed
    state idle
    state idle1
      en:
      oMdReq = true;
    (default) -> idle
    idle -> idle1 : [after(iLongPressThrshhldTm,tick)]
  (default) -> NotPressed : {oMdInterruptCnt = 0;}
  NotPressed -> NotPressed [order 1] : [(iSRSMode != SRSMode1.SRSSlctSwStat_None) &&...
      | hasChangedTo(iCnfmSwReq, true)]
      | {oMdInterruptCnt ++;}
  NotPressed -> ButtonPressed [order 2] : [iCurMdState == MdTp1.MdTp_None &&...
      | hasChangedTo(iSrc, true)]
  ButtonPressed -> NotPressed : [!iSrc]
  data: iSrc input boolean; oMdReq output boolean; oMdInterruptCnt output uint8; iLongPressThrshhldTm input uint8; iCurMdState input Enum: MdTp1; iCmpReq input; iCnfmSwReq input boolean; iSRSMode input Enum: SRSCurMode1

== stateflow chart ModeInputHandle/ModelInputHandleRunnable_sys/Subsystem1/VipMdReq/ButtonLongPressed/Chart1 ==
  state NotPressed
    en:
    oMdReq = false;
  state ButtonPressed
    state idle
      en:
      oMdInterruptCnt ++;
    state idle1
      en:
      oMdReq=true;
    (default) -> idle
    idle -> idle1 [order 1] : [after(iLongPressThrshhldTm,tick)]
  state wait
    en:
    oMdReq = false;
  (default) -> NotPressed : {oMdInterruptCnt = 0;}
  NotPressed -> ButtonPressed : [hasChangedTo(iSrc, true)]
  idle -> NotPressed [order 2] : [!iSrc]
  wait -> NotPressed : [!iSrc]
  idle1 -> wait [order 2] : //[after(5,tick)]
      | [after(2,tick)]
  idle1 -> NotPressed [order 1] : [!iSrc]
  data: iSrc input boolean; oMdReq output boolean; oMdInterruptCnt output uint8; iLongPressThrshhldTm input uint8

== stateflow chart ModeInputHandle/ModelInputHandleRunnable_sys/Subsystem1/VipMdReq/ButtonLongPressed1/Chart1 ==
  state NotPressed
    en:
    oMdReq = false;
  state ButtonPressed
    state idle
      en:
      oMdInterruptCnt ++;
    state idle1
      en:
      oMdReq=true;
    (default) -> idle
    idle -> idle1 [order 1] : [after(iLongPressThrshhldTm,tick)]
  state wait
    en:
    oMdReq = false;
  (default) -> NotPressed : {oMdInterruptCnt = 0;}
  NotPressed -> ButtonPressed : [hasChangedTo(iSrc, true)]
  idle -> NotPressed [order 2] : [!iSrc]
  wait -> NotPressed : [!iSrc]
  idle1 -> wait [order 2] : //[after(5,tick)]
      | [after(2,tick)]
  idle1 -> NotPressed [order 1] : [!iSrc]
  data: iSrc input boolean; oMdReq output boolean; oMdInterruptCnt output uint8; iLongPressThrshhldTm input uint8

== stateflow chart ModeInputHandle/ModelInputHandleRunnable_sys/Subsystem1/VipMdReq/ButtonLongPressed2/Chart1 ==
  state NotPressed
    en:
    oMdReq = false;
  state ButtonPressed
    state idle
    state idle1
      en:
      oMdReq = true;
    (default) -> idle
    idle -> idle1 : [after(iLongPressThrshhldTm,tick)]
  (default) -> NotPressed : {oMdInterruptCnt = 0;}
  NotPressed -> NotPressed [order 1] : [(iSRSMode != SRSCurMode1.SRSMode_None) &&...
      | hasChangedTo(iCnfmSwReq, true)]
      | {oMdInterruptCnt ++;}
  NotPressed -> ButtonPressed [order 2] : [iCurMdState == MdTp1.MdTp_None &&...
      | hasChangedTo(iSrc, true)]
  ButtonPressed -> NotPressed : [!iSrc]
  data: iSrc input boolean; oMdReq output boolean; oMdInterruptCnt output uint8; iLongPressThrshhldTm input uint8; iCurMdState input Enum: MdTp1; iCmpReq input; iCnfmSwReq input boolean; iSRSMode input Enum: SRSCurMode1

== stateflow chart ModeInputHandle/ModelInputHandleRunnable_sys/Subsystem1/VipMdReq/ButtonLongPressed3/Chart1 ==
  state NotPressed
    en:
    oMdReq = false;
  state ButtonPressed
    state idle
    state idle1
      en:
      oMdReq = true;
    (default) -> idle
    idle -> idle1 : [after(iLongPressThrshhldTm,tick)]
  (default) -> NotPressed : {oMdInterruptCnt = 0;}
  NotPressed -> NotPressed [order 1] : [(iSRSMode != SRSCurMode1.SRSMode_None) &&...
      | hasChangedTo(iCnfmSwReq, true)]
      | {oMdInterruptCnt ++;}
  NotPressed -> ButtonPressed [order 2] : [iCurMdState == MdTp1.MdTp_None &&...
      | hasChangedTo(iSrc, true)]
  ButtonPressed -> NotPressed : [!iSrc]
  data: iSrc input boolean; oMdReq output boolean; oMdInterruptCnt output uint8; iLongPressThrshhldTm input uint8; iCurMdState input Enum: MdTp1; iCmpReq input; iCnfmSwReq input boolean; iSRSMode input Enum: SRSCurMode1

== stateflow chart ModeInputHandle/ModelInputHandleRunnable_sys/Subsystem1/VipMdReq/ButtonLongPressed4/Chart1 ==
  state NotPressed
    en:
    oMdReq = false;
  state ButtonPressed
    state idle
    state idle1
      en:
      oMdReq = true;
    (default) -> idle
    idle -> idle1 : [after(iLongPressThrshhldTm,tick)]
  (default) -> NotPressed : {oMdInterruptCnt = 0;}
  NotPressed -> NotPressed [order 1] : [(iSRSMode != SRSCurMode1.SRSMode_None) &&...
      | hasChangedTo(iCnfmSwReq, true)]
      | {oMdInterruptCnt ++;}
  NotPressed -> ButtonPressed [order 2] : [iCurMdState == MdTp1.MdTp_None &&...
      | hasChangedTo(iSrc, true)]
  ButtonPressed -> NotPressed : [!iSrc]
  data: iSrc input boolean; oMdReq output boolean; oMdInterruptCnt output uint8; iLongPressThrshhldTm input uint8; iCurMdState input Enum: MdTp1; iCmpReq input; iCnfmSwReq input boolean; iSRSMode input Enum: SRSCurMode1
